simulink model "example_FanMain"  (R2018b)
settings: Solver=VariableStepAuto  StartTime=0.0  StopTime=240  RelTol=1e-3
undefined symbols (not defined in the file): density, Fan_Const, ID, MassFlow, path_carnot, Pressure, Temperature, Water
libraries: carnot x8
settings Model: Creator=drhf  LastModifiedBy=drhf

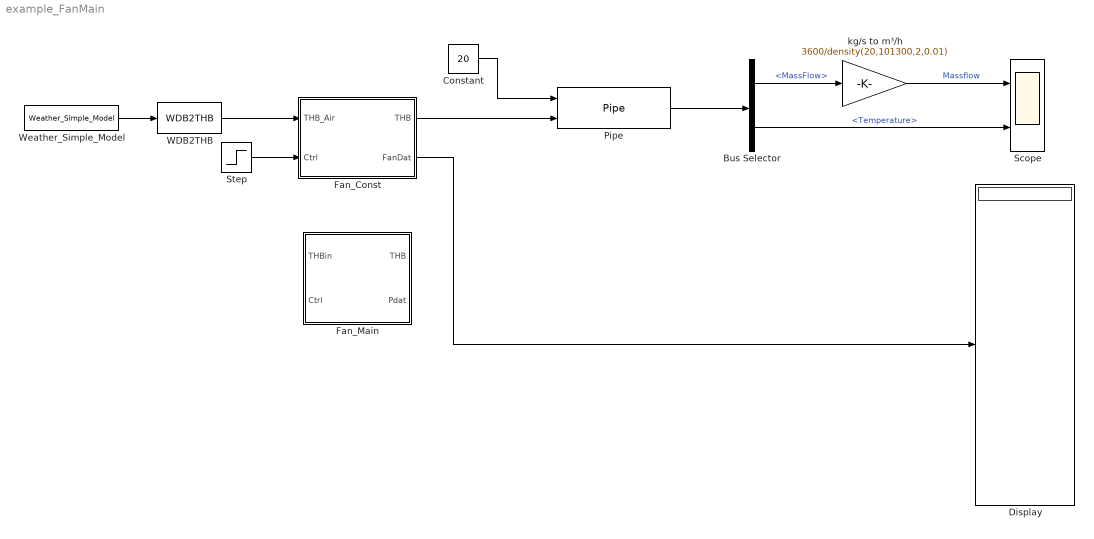
== system example_FanMain ==
  Bus Selector : BusSelector  OutputSignals=MassFlow,Temperature
  Constant : Constant  Value=20
  Display : Display
  Fan_Const : Subsystem  AncestorBlock=Fan_Const/Fan_Const  mask(Fan constant){Vdotmax=1000, dia=0.02, p0=101300, mix=0.01, Tini=20, UA=3, mcp=1000, e0=10, e1=10, e2=-1}
      mask prompts: Vdotmax "Vdotmax : volume flowrate in m³/h"; dia "diameter at in- and outlet [m]"; p0 "air pressure in Pa"; mix "kg of water per kg of dry air"; Tini "ambient and start temperature in °C"; UA "Thermal loss coefficient to ambient in W/K"; mcp "mcp: thermal capacity of the node in J/K"; e0 "e0: constant coefficient in W"; e1 "e1: linear coefficient in W*s/kg"; e2 "e2: quadratic coefficient in W*(s/kg)²"
      mask help:
      | Set constant volume flowrate according to the parameter Vdotmax and the control signal:
      | mdot = Vdotmax * Ctrl
      | Keep in mind that the flowrate in the THB is the massflowrate in kg/s whereas the parameters of the fan have different units.
      | Use the option "thermal node" if you want the pump to have thermal capacity and losses to ambient (or if you want to break an algebraic loop in the temperature signal).
      | Electric power is calculated Pel = e0 + e1*mdot + e2*mdot^2
      mask Help: web(fullfile(path_carnot('help'),'Pump_Const.html'),'-helpbrowser')
      mask TypeOptions dia: Pump_Const/dia
      mask TypeOptions mix: Pump_Const/mix
      mask TypeOptions Tini: Pump_Const/Tini
      mask TypeOptions UA: Pump_Const/UA
      mask TypeOptions mcp: Pump_Const/mcp
      mask TypeOptions e0: Pump_Const/e0
      mask TypeOptions e1: Pump_Const/e1
      mask TypeOptions e2: Pump_Const/e2
      mask DialogControl ParameterTabVar0 Prompt: Hydraulic
      mask DialogControl Container7 Prompt: Initial Values
      mask DialogControl ParameterTabVar012 Prompt: Thermal
      mask DialogControl ParameterTabVar01 Prompt: Electric
      mask Display:
      | plot(0,0,100,100,...
      |     [40,70,40,30,30,40,60,70,70,60,40],[70,50,30,40,60,70,70,60,40,30,30])
  Fan_Main : Subsystem  mask(Pump Main){Tini=20, p0=3e5, IDpreset=pressure drop, fluid=Water, mix=0, mix2=0, mix3=0, t1=1, PathName=fullfile(path_carnot('libsl'), 'Hydraulics', 'Pump_Main', 'parameter_set'), FileName='Pump6m.mat', userPath=off, userParam=off, a0=60000, a1=-43200, a2=0, dia=0.025, UA=1, mcp=4182, e0=50, e1=28.8, e2=-10.368}
      mask prompts: Tini "Ambient temperature for losses and initial temperture in °C"; p0 "System pressure at pump inlet [Pa]"; IDpreset "Pressure calculation"; mix "Fluid mixture    [0..1]"; mix2 "Fluid mixture 2 [0..1]"; mix3 "Fluid mixture 3 [0..1]"; t1 "Time constant [s] of PT1 transfer function for massflow"; PathName "Path"; FileName "Parameter set"; userPath "Edit path and name of parameter set"; userParam "User defined parameters"; a0 "a0: pump head in [Pa] (pressure increase at zero flow)"; a1 "a1: pump characteristic linear coefficient [Pa*s/kg]"; a2 "a2: pump characteristic quadratic coefficient [Pa*(s/kg)²]"; dia "Diameter at in- and outlet [m]"; UA "UA: thermal loss coefficient in W/K"; mcp "mcp: thermal capacity of the node in J/K"; e0 "e0: constant coefficient in W"; e1 "e1: linear coefficient in W*s/kg"; e2 "e2: quadratic coefficient in W*(s/kg)²"
      mask help:
      | This is the main pump in a circuit. Every circuit must have exactly ONE 'Pump_Main'. Use the 'Pump_Additional' blocks if you want to use more pumps.
      | The Pump_Main calculate massflow by setting pressure drop in the circuit (dp_circuit) equal to the pressure increase of the pump (dp_pump).
      |   dp_circuit = c + l*mdot + q*mdot²
      |   dp_pump_ = a0*Ctrl + a1*mdot +a2*mdot²
      | with
      |   mdot : massflow in kg/s
      |   Ctrl : Control signal input [0..1]
      mask init:
      | % callback to set parameters of model
      | [ok, param] = CarnotCallbacks_PumpMain('SetParameters',gcbh,PathName,FileName);
      mask Help: web(fullfile(path_carnot('help'),'Pump_Main.html'),'-helpbrowser')
      mask TypeOptions Tini: ThermalNodeTHB/Tini
      mask TypeOptions p0: basic_THB/p
      mask TypeOptions IDpreset: ID/IDpreset
      mask TypeOptions fluid: basic_THB/fluid
      mask TypeOptions mix: basic_THB/mix
      mask TypeOptions mix2: basic_THB/mix2
      mask TypeOptions mix3: basic_THB/mix3
      mask TypeOptions t1: Transfer Fcn/t1
      mask Callback userPath: [ok, param] = CarnotCallbacks_PumpMain('UserEdit',gcbh);
      mask Callback userParam: [ok, param] = CarnotCallbacks_PumpMain('UserEdit',gcbh);
      mask TypeOptions a0: PumpHead/Gain
      mask TypeOptions a1: PumpLinear/Value
      mask TypeOptions a2: PumpQuadratic/Value
      mask TypeOptions dia: basic_THB/dia
      mask TypeOptions UA: ThermalNodeTHB/UA
      mask TypeOptions mcp: ThermalNodeTHB/mcp
      mask TypeOptions e0: ElectricConsumptionPump/e0
      mask TypeOptions e1: ElectricConsumptionPump/e1
      mask TypeOptions e2: ElectricConsumptionPump/e2
      mask DialogControl ParameterGroupFile Prompt: Picking a parameter set
      mask DialogControl Control1 Prompt: Carnot public data
      mask DialogControl Control1 Callback: [ok, file] = CarnotCallbacks_PumpMain('GetFilename',gcbh,'public');
      mask DialogControl Control3 Prompt: Carnot internal data
      mask DialogControl Control3 Callback: [ok, file] = CarnotCallbacks_PumpMain('GetFilename',gcbh,'internal');
      mask DialogControl Control4 Prompt: Selected path
      mask DialogControl Control4 Callback: [ok, file] = CarnotCallbacks_PumpMain('GetFilename',gcbh,'selected');
      mask DialogControl PrameterGroupUser Prompt: Parameter Values
      mask DialogControl Container9 Prompt: Hydraulic
      mask DialogControl Container7 Prompt: Thermal
      mask DialogControl Control9 Prompt: Thermal node for temperature:  mcp * dTnode/dt = UA*(Tamb-Tnode) + mdot*cp_in*(Tin-Tnode)
      mask DialogControl Container14 Prompt: Electric
      mask DialogControl Control7 Prompt: Power consumption  Pel = e0 + e1*mdot + e2*mdot²
      mask DialogControl Control5 Prompt: Save in Carnot internal data
      mask DialogControl Control5 Callback: [ok, param] = CarnotCallbacks_PumpMain('SaveFilename',gcbh,'internal','B');
      mask DialogControl Control6 Prompt: Save in selected path
      mask DialogControl Control6 Callback: [ok, param] = CarnotCallbacks_PumpMain('SaveFilename',gcbh,'selected','B');
      mask Display:
      | % user defined picture file
      | picfile = fullfile(path_carnot('intlibsl'), ...
      |         'Hydraulics', 'Pump_Main', 'PumpMain.jpg');
      | 
      | pic = false;
      | if ~BlockIsInCarnotLibrary    % if not located in library any more
      |     if exist(picfile,'file') % show internal picture if defined
      |         image(imread(picfile), [0.2, 0, 0.6, 1])
      |         set_param(gcb, 'BackgroundColor', 'White')
      |         pic = true;
      |     end
      | end
      | if ~pic    % show public picture
      |     set_param(gcb, 'BackgroundColor', 'green')
      |     plot(0,0,1,1,[40,70,40,30,30,40,60,70,70,60,40]/100, ...
      |         [70,50,30,40,60,70,70,60,40,30,30]/100)
      |     disp('main')
      | end
  Pipe : carnot/Hydraulics/Pipe  dia=0.3  len=10  hgt=0  uloss=100/20/10  cond=0  cwall=1000  t0=20  lin=100/0.2  qua=100/0.2^2  nodes=10
      settings: SourceProductName=Carnot
  Scope : Scope  NumInputPorts=2
  Step : Step  Time=120  SampleTime=0
  WDB2THB : carnot/Weather/WDB2THB  dia=0.2
      settings: SourceProductName=Carnot
  Weather_Simple_Model : carnot/Weather/Weather_Simple_Model  Ibn=900  Idg=100  tamb=5  deltaTsky=-6  rh=50  precip="10e-3/24/3600           % 10 mm in 24 h"  cloud=0.125  p=1013e2  vw=1  wdir=270  lat=60  colangle=0  colazi=0  colrot=0
      settings: SourceProductName=Carnot
  kg/s to m³/h : Gain  Gain=3600/density(20,101300,2,0.01)
  wires:
  Weather_Simple_Model/1 -> WDB2THB/1
  Step/1 -> Fan_Const/2(Ctrl)
  Fan_Const/1(THB) -> Pipe/2
  Constant/1 -> Pipe/1
  Fan_Const/2(FanDat) -> Display/1
  Pipe/1 -> Bus Selector/1
  Bus Selector/1 -> kg/s to m³/h/1  "<MassFlow>"
  kg/s to m³/h/1 -> Scope/1  "Massflow"
  WDB2THB/1 -> Fan_Const/1(THB_Air)
  Bus Selector/2 -> Scope/2  "<Temperature>"

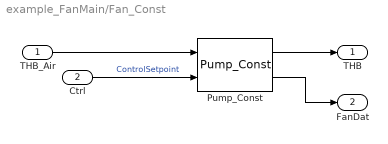
== system example_FanMain/Fan_Const ==
  THB_Air : Inport
  Ctrl : Inport  Port=2
  Pump_Const : carnot/Hydraulics/Pump_Const  mdotmax=Vdotmax/3600*density(Tini,p0,2,0)  dia=dia  p0=p0  fluid_id=Air  mix=mix  mix2=0  mix3=0  UA=UA  mcp=mcp  Tini=Tini  e0=e0  e1=e1  e2=e2
      settings: SourceProductName=Carnot
  THB : Outport
  FanDat : Outport  Port=2
  wires:
  THB_Air/1 -> Pump_Const/1
  Ctrl/1 -> Pump_Const/2  "ControlSetpoint"
  Pump_Const/1 -> THB/1
  Pump_Const/2 -> FanDat/1

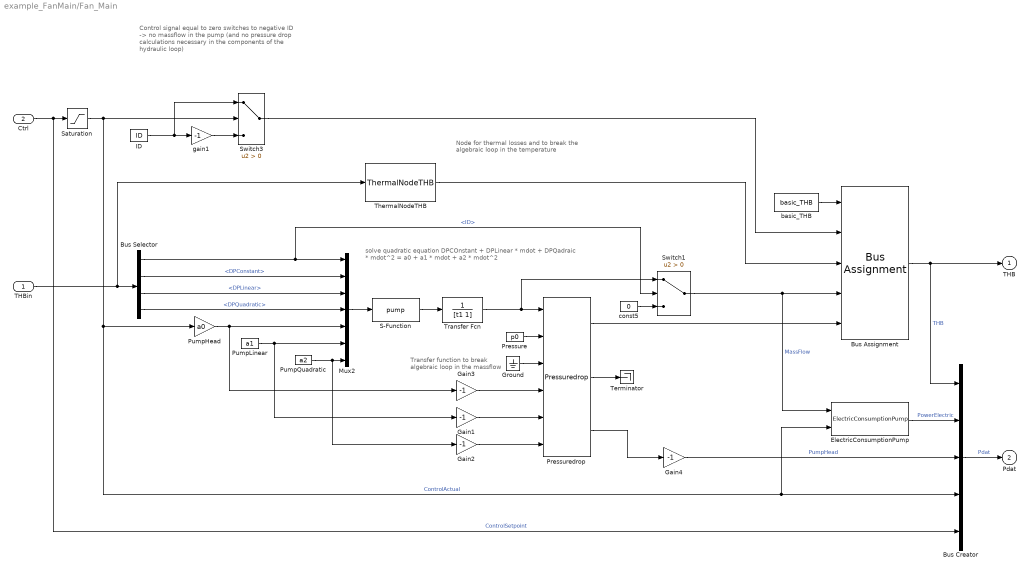
== system example_FanMain/Fan_Main ==
  note: Node for thermal losses and to break
      | the algebraic loop in the temperature
  note: Transfer function to
      | break algebraic loop
      | in the massflow
  note: solve quadratic equation
      | DPCOnstant + DPLinear * mdot + DPQadraic * mdot^2
      | = a0 + a1 * mdot + a2 * mdot^2
  note: Control signal equal to zero switches
      | to negative ID -> no massflow in the
      | pump (and no pressure drop calculations
      | necessary in the components of the
      | hydraulic loop)
  THBin : Inport
  Ctrl : Inport  Port=2
  Bus Assignment : BusAssignment  AssignedSignals=ID,Temperature,MassFlow,Pressure
  Bus Creator : BusCreator  Inputs=5
  Bus Selector : BusSelector  OutputSignals=ID,DPConstant,DPLinear,DPQuadratic
  ElectricConsumptionPump : carnot/Basic/Hydraulics/ElectricConsumptionPump  e0=e0  e1=e1  e2=e2
      settings: SourceProductName=Carnot
  Gain{1..4} (4 alike) : Gain  Gain=-1
  Ground : Ground
  ID : Constant  Value=ID  mask{IDpreset=pressure drop}
      mask prompts: IDpreset "Calculation"
      mask init:
      | ID = IDpreset*10000 + 1;
      mask TypeOptions IDpreset: pressure drop | pressure drop and pressure head
  Mux2 : Mux  Inputs=7
  Pressure : Constant  Value=p0
  Pressuredrop : carnot/Basic/Pressure_Drop/Pressuredrop
      settings: SourceProductName=Carnot
  PumpHead : Gain  Gain=a0
  PumpLinear : Constant  Value=a1
  PumpQuadratic : Constant  Value=a2
  S-Function : S-Function  FunctionName=pump  SFunctionDeploymentMode=off  EnableBusSupport=off
  Saturation : Saturate  UpperLimit=1  LowerLimit=0
  Switch1 : Switch  Criteria=u2 > Threshold  SaturateOnIntegerOverflow=on  InputSameDT=on
  Switch3 : Switch  Criteria=u2 > Threshold  SaturateOnIntegerOverflow=on  InputSameDT=on
  Terminator : Terminator
  ThermalNodeTHB : carnot/Basic/Thermal_Models/ThermalNodeTHB  UA=UA  mcp=mcp  Tini=Tini
      settings: SourceProductName=Carnot
  Transfer Fcn : TransferFcn  Denominator=[t1 1]  mask{t1=t1}
      mask prompts: t1 "Time constant of PT1 transfer function for massflow in s"
  basic_THB : carnot/Basic/Hydraulics/basic_THB  t=20  mdot=0  p=p0  ID=No Pressure Drop  fluid=Water  mix=mix  mix2=mix2  mix3=mix3  dia=dia  hgt=0
      settings: SourceProductName=Carnot
  const5 : Constant  Value=0
  gain1 : Gain  Gain=-1  SaturateOnIntegerOverflow=on  OutDataTypeStr=Inherit: Same as input  ParamDataTypeStr=Inherit: Same as input
  THB : Outport
  Pdat : Outport  Port=2
  wires:
  ElectricConsumptionPump/1 -> Bus Creator/2  "PowerElectric"
  Bus Creator/1 -> Pdat/1  "Pdat"
  THBin/1 -> Bus Selector/1, ThermalNodeTHB/1
  Pressuredrop/3 -> Gain4/1
  Bus Selector/1 -> Switch1/2, Mux2/1  "<ID>"
  Switch1/1 -> Bus Assignment/4, ElectricConsumptionPump/1  "MassFlow"
  Mux2/1 -> S-Function/1
  S-Function/1 -> Transfer Fcn/1
  PumpLinear/1 -> Gain1/1, Mux2/6
  PumpQuadratic/1 -> Gain2/1, Mux2/7
  PumpHead/1 -> Gain3/1, Mux2/5
  Ctrl/1 -> Saturation/1, Bus Creator/5  "ControlSetpoint"
  ID/1 -> Switch3/1, gain1/1
  gain1/1 -> Switch3/3
  Transfer Fcn/1 -> Pressuredrop/1, Switch1/1
  const5/1 -> Switch1/3
  basic_THB/1 -> Bus Assignment/1
  Bus Assignment/1 -> THB/1, Bus Creator/1  "THB"
  Switch3/1 -> Bus Assignment/2
  ThermalNodeTHB/1 -> Bus Assignment/3
  Bus Selector/2 -> Mux2/2  "<DPConstant>"
  Bus Selector/3 -> Mux2/3  "<DPLinear>"
  Bus Selector/4 -> Mux2/4  "<DPQuadratic>"
  Pressure/1 -> Pressuredrop/2
  Pressuredrop/1 -> Bus Assignment/5
  Ground/1 -> Pressuredrop/3
  Pressuredrop/2 -> Terminator/1
  Saturation/1 -> Switch3/2, PumpHead/1, ElectricConsumptionPump/2, Bus Creator/4  "ControlActual"
  Gain3/1 -> Pressuredrop/4
  Gain1/1 -> Pressuredrop/5
  Gain2/1 -> Pressuredrop/6
  Gain4/1 -> Bus Creator/3  "PumpHead"
